simulink model "obserwator_pelnego_rzedu"  (R2018b)
settings: Solver=VariableStepAuto  StartTime=0.0  StopTime=10  RelTol=1e-3
values from neighbouring files (symbols this model uses):
  K_x = K_9    [zad5.m]
  L_x = L_6    [zad7.m]
undefined symbols (not defined in the file or in its folder): A, C
settings Model: Creator=mariu  LastModifiedBy=mariu

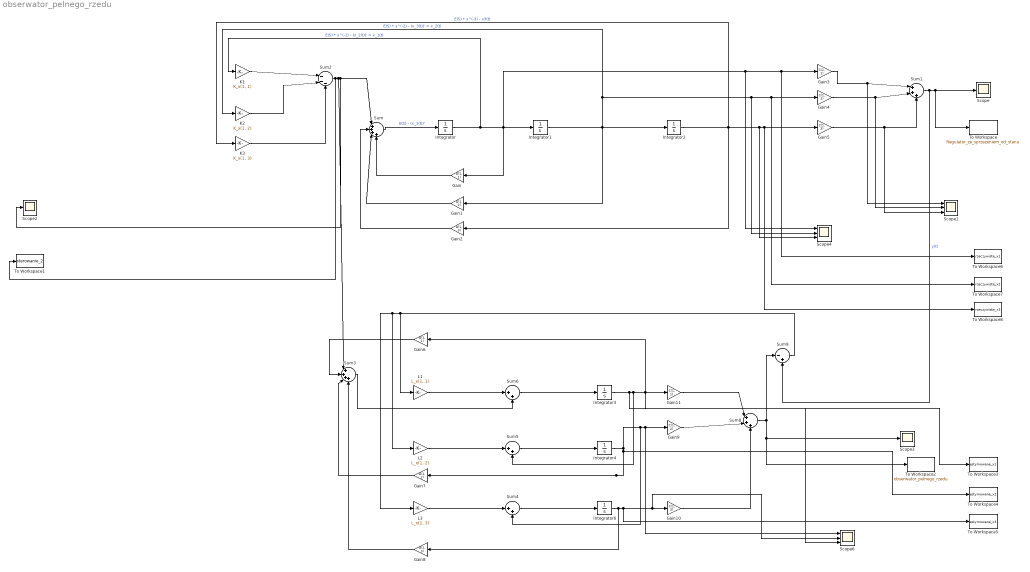
== system obserwator_pelnego_rzedu ==
  Gain : Gain  Gain=A(1, 1)
  Gain1 : Gain  Gain=A(1, 2)
  Gain10 : Gain  Gain=C(1, 3)
  Gain11 : Gain  Gain=C(1, 1)
  Gain2 : Gain  Gain=A(1, 3)
  Gain3 : Gain  Gain=C(1, 1)
  Gain4 : Gain  Gain=C(1, 2)
  Gain5 : Gain  Gain=C(1, 3)
  Gain6 : Gain  Gain=A(1, 1)
  Gain7 : Gain  Gain=A(1, 2)
  Gain8 : Gain  Gain=A(1, 3)
  Gain9 : Gain  Gain=C(1, 2)
  Integrator : Integrator  InitialCondition=-1
  Integrator1 : Integrator  InitialCondition=2
  Integrator2 : Integrator  InitialCondition=1
  Integrator3 : Integrator
  Integrator4 : Integrator
  Integrator6 : Integrator
  "K1 " : Gain  Gain=K_x(1, 1)
  "K2 " : Gain  Gain=K_x(1, 2)
  "K3 " : Gain  Gain=K_x(1, 3)
  "L1 " : Gain  Gain=L_x(1, 1)
  "L2 " : Gain  Gain=L_x(1, 2)
  "L3 " : Gain  Gain=L_x(1, 3)
  Scope : Scope
  Scope1 : Scope  NumInputPorts=3
  Scope2 : Scope
  Scope3 : Scope
  Scope4 : Scope  NumInputPorts=3
  Scope6 : Scope  NumInputPorts=3
  Sum : Sum  Inputs=|++++
      settings: AttributesFormatString=%<Inputs>
  Sum1 : Sum  Inputs=|+++
      settings: AttributesFormatString=%<Inputs>
  Sum2 : Sum  Inputs=|---
      settings: AttributesFormatString=%<Inputs>
  Sum3 : Sum  Inputs=|++++
      settings: AttributesFormatString=%<Inputs>
  Sum4 : Sum  Inputs=|++
      settings: AttributesFormatString=%<Inputs>
  Sum5 : Sum  Inputs=|++
      settings: AttributesFormatString=%<Inputs>
  Sum6 : Sum  Inputs=|++
      settings: AttributesFormatString=%<Inputs>
  Sum8 : Sum  Inputs=|+++
      settings: AttributesFormatString=%<Inputs>
  Sum9 : Sum  Inputs=|-+
      settings: AttributesFormatString=%<Inputs>
  To Workspace : ToWorkspace  VariableName=Regulator_ze_sprzezeniem_od_stanu  SaveFormat=Timeseries  SampleTime=-1
  To Workspace1 : ToWorkspace  VariableName=sterowanie_2  SaveFormat=Timeseries  SampleTime=-1
  To Workspace2 : ToWorkspace  VariableName=obserwator_pelnego_rzedu  SaveFormat=Timeseries  SampleTime=-1
  To Workspace3 : ToWorkspace  VariableName=estymowane_x1  SaveFormat=Timeseries  SampleTime=-1
  To Workspace4 : ToWorkspace  VariableName=estymowane_x2  SaveFormat=Timeseries  SampleTime=-1
  To Workspace5 : ToWorkspace  VariableName=estymowane_x3  SaveFormat=Timeseries  SampleTime=-1
  To Workspace6 : ToWorkspace  VariableName=rzeczywiste_x1  SaveFormat=Timeseries  SampleTime=-1
  To Workspace7 : ToWorkspace  VariableName=rzeczywiste_x2  SaveFormat=Timeseries  SampleTime=-1
  To Workspace8 : ToWorkspace  VariableName=rzeczywiste_x3  SaveFormat=Timeseries  SampleTime=-1
  wires:
  Sum1/1 -> Sum9/2, To Workspace/1, Scope/1  "y(t)"
  Integrator1/1 -> "K2 "/1, Scope4/2, To Workspace7/1, Gain4/1, Gain1/1, Integrator2/1  "E(S) * s^(-2) - (x_3(t))' = x_2(t)"
  Gain3/1 -> Scope1/1, Sum1/1
  Integrator/1 -> "K1 "/1, Scope4/1, To Workspace6/1, Gain3/1, Gain/1, Integrator1/1  "E(S) * s^(-1) - (x_2(t))' = x_1(t)"
  Gain5/1 -> Scope1/3, Sum1/3
  Sum/1 -> Integrator/1  "E(S) - (x_1(t))'"
  Integrator2/1 -> Gain2/1, "K3 "/1, Scope4/3, To Workspace8/1, Gain5/1  "E(S) * s^(-3) - x3(t)"
  Gain4/1 -> Scope1/2, Sum1/2
  Gain1/1 -> Sum/3
  Gain/1 -> Sum/4
  Gain2/1 -> Sum/2
  "K2 "/1 -> Sum2/2
  "K1 "/1 -> Sum2/1
  "K3 "/1 -> Sum2/3
  Sum2/1 -> To Workspace1/1, Sum/1, Scope2/1, Sum3/1
  Sum6/1 -> Integrator3/1
  Sum4/1 -> Integrator6/1
  Integrator3/1 -> To Workspace3/1, Scope6/3, Gain6/1, Gain11/1, Sum5/2
  Integrator4/1 -> To Workspace4/1, Gain7/1, Sum4/2, Scope6/1, Gain9/1
  Integrator6/1 -> To Workspace5/1, Scope6/2, Gain10/1, Gain8/1
  Sum5/1 -> Integrator4/1
  "L1 "/1 -> Sum6/1
  "L2 "/1 -> Sum5/1
  "L3 "/1 -> Sum4/1
  Gain6/1 -> Sum3/2
  Gain7/1 -> Sum3/3
  Sum9/1 -> "L3 "/1, "L2 "/1, "L1 "/1
  Gain8/1 -> Sum3/4
  Gain9/1 -> Sum8/2
  Gain11/1 -> Sum8/1
  Gain10/1 -> Sum8/3
  Sum8/1 -> Sum9/1, Scope3/1, To Workspace2/1
  Sum3/1 -> Sum6/2
